simulink model "Validation_Tricopter_Model"  (R2015a)
settings: Solver=ode3  SolverMode=SingleTasking  StartTime=0.0  StopTime=20  FixedStep=T_sim  RelTol=1e-3
PreLoadFcn:
  | LoadLibraries
values from neighbouring files (symbols this model uses):
  a = 10.26    [SetupComplete.m]
  A_x = 0.015    [SetupComplete.m]
  A_y = A_x    (= 0.015)    [SetupComplete.m]
  A_z = 0.16    [SetupComplete.m]
  C_d0 = 0.001193    [SetupComplete.m]
  C_x = 1.2    [SetupComplete.m]
  C_y = C_x    (= 1.2)    [SetupComplete.m]
  C_z = 2.2    [SetupComplete.m]
  CG_0 = [0,0,0.02]'    [SetupComplete.m]
  g = 9.81    [SetupComplete.m]
  h = 0.08    [SetupComplete.m]
  h_FA = 0.02    [SetupComplete.m]
  h_M = 0.064    [SetupComplete.m]
  I_BAC_0 = [ Ix,0,Ixz;0,Iy,0;Ixz,0,Iz]    [SetupComplete.m]
  I_prop = 1/4*M_eq*R^2*diag([1,1,2])    [SetupComplete.m]
  I_tube = [1/2*M_tube*R_tube_eq^2,0,  0  ;           0 ,1/3*M_tube*l_arm^2,0;             0  ,0,1/3*M_tube*l_arm^2]    [SetupComplete.m]
  Initial_Omegas = [1;1;1]*Omega_hover    [Run3Copter.m]
  J_FA = I_prop(1,1) + m_prop*h^2  + m_FA*h_FA^2 + m_M*h_M^2    [SetupComplete.m]
  J_T = J_m+1/2*M_eq*R^2    (= 2.000642e-05)    [SetupComplete.m]
  Ki = lqi(LM_4DOF_aug, Q,R)    [robust_controller.m]
  l = 0.3450    (= 0.345)    [NDI_components.m]    (also in SetupComplete.m; robust_controller.m)
  l_arm = 0.264    [SetupComplete.m]
  m = 3.51    [SetupComplete.m]
  m_0 = 2.61    [SetupComplete.m]
  m_FA = 0.02    [SetupComplete.m]
  m_M = 0.300    (= 0.3)    [SetupComplete.m]
  m_prop = 0.02    [SetupComplete.m]
  R = 0.1778    [SetupComplete.m]    (also in robust_controller.m = eye(4))
  rho = 1.15    [SetupComplete.m]
  sigma = b*c/(pi*R)    (= 0.107416159567)    [SetupComplete.m]
  T_sim = 0.01    [Run3Copter.m]
  theta_0 = 0.38397    [SetupComplete.m]
  theta_1 = -0.2967    [SetupComplete.m]
  trim_simplemodel = [0.589627915568 -2.20656039197 0 0.588313336084 0 0 0.588313330414 0 0]    [trimvalues.mat]
  V_4DOF_last = [0.0122475086001 0.00870447045314 -0.0292257707267 -0.0198753669721 -0.00290766514824 -0.0269511839788 0.0344308792695 -0.0305235710433 -0.0274078219028 -0.0329291952852 -0.0272335702183 -0.00643013158961 ... (1500 elements, 50x30)]    [NN_c_weights.mat]
  v_i0 = sqrt( 1/3*m*g/(2*rho*pi*R^2)  )    [SetupComplete.m]
  W_4DOF_last = [0.0132359246225 -0.0402459595001 -0.0221501781133 0.0046881519205 0.0457506835434 0.0464888535199 -0.0342386918322 0.0470592781761 0.0457166948243 -0.00146243512772 0.0300280468889 -0.0358113661373 ... (204 elements, 4x51)]    [NN_c_weights.mat]
undefined symbols (not defined in the file or in its folder): DOWN_0, EAST_0, Motor, NORTH_0, P_0, Prop, Q_0, R_0, sigmatest, U_0, V_0, v_i_adim, Vx_adim, Vz_adim, W_0
undefined symbols (not defined in the file): Initial_Torques, Rotation_sign, Tau_motors
libraries: simulink x66, XXCopter x32, vrlib x26, simulink_extras x6, Adaptive_FaultTolerantControl x6, qcatlib x4, dspinverses x4, lib_controller x4, aerolib6dofsys x3, aerolibtransform2 x3, aerolib6dof2 x1
(part 11 of 11)

== matlab function Validation_Tricopter_Model/3 Copter Complete/Arms Dynamics: Forces and Moments/4 DOF Arms Dynamics: Forces and Moments1/4 DOF Arms Dynamics: Forces and Moments1/Arm Dynamics/Gyroscopic Moments/Arm Inertia1 ==
  data: T_FAFb input; Arm_axis input; J_Arm output; I_tube parameter; I_prop parameter; h_FA parameter; h_M parameter; m_FA parameter; m_M parameter; m_prop parameter; h parameter
function J_Arm  = Arm_inertia(T_FAFb,Arm_axis, I_tube, I_prop, h_FA, h_M, m_FA, m_M, m_prop, h)


r_FAO=Arm_axis+T_FAFb*[0;0;-h_FA];
r_MO=Arm_axis+T_FAFb*[0;0;-h_M];
r_po=Arm_axis+T_FAFb*[0;0;-h];

I_FA = m_FA*[ r_FAO(2)^2+r_FAO(3)^2,r_FAO(1)*r_FAO(2),r_FAO(1)*r_FAO(3);...
            r_FAO(1)*r_FAO(2), r_FAO(1)^2+r_FAO(3)^2, r_FAO(2)*r_FAO(3);...
            r_FAO(1)*r_FAO(3),r_FAO(2)*r_FAO(3), r_FAO(1)^2+r_FAO(2)^2];
I_M = m_M*[ r_MO(2)^2+r_MO(3)^2,r_MO(1)*r_MO(2),r_MO(1)*r_MO(3);...
            r_MO(1)*r_MO(2), r_MO(1)^2+r_MO(3)^2, r_MO(2)*r_MO(3);...
            r_MO(1)*r_MO(3),r_MO(2)*r_MO(3), r_MO(1)^2+r_MO(2)^2];
I_steiner = m_prop*[ r_po(2)^2+r_po(3)^2,r_po(1)*r_po(2),r_po(1)*r_po(3);...
            r_po(1)*r_po(2), r_po(1)^2+r_po(3)^2, r_po(2)*r_po(3);...
            r_po(1)*r_po(3),r_po(2)*r_po(3), r_po(1)^2+r_po(2)^2];


% J_Arm = T_FAFb*I_prop*T_FAFb'+ I_tube +I_FA+I_M+I_steiner;
J_Arm = T_FAFb*I_prop*T_FAFb' +I_FA+I_M+I_steiner; % Quitamos el tubo ya que es insignificante y hay que calcularlo para cada brazo

== matlab function Validation_Tricopter_Model/Controller/NDI+CA Controller/4DOF ANN+NDI+CA Controller - No massic update/G(X) 4DOF_WPQR ==
  data: gx output size=[4,4]; prev_input input size=[9,1]
function gx = gx(prev_input)
    % Calculates f_hat(x). The expression is calculated in NDI_components
    % x_dot = f(x) + g(x,u)
    %   g(x,u) ~= g(x,u0) + jac(g(x,u), u)(u0) * (u - u0)
    %   g(x,u) ~= h(x,u0) + jac(g(x,u), u)(u0) * u
    % x_dot = f_hat(x) + jac(g(x,u), u) * u
    %   f_hat(x) = f(x) + g(x,u0) - jac(g(x,u), u)(u0) *  u0
    %   g_hat(x) = jac(g(x,u), u)(u0)
    % x_dot = f_hat(x) + g_hat(x) * u
    tau1_0 = prev_input(1);
    eta1_0 = prev_input(2);
    gamma1_0 = prev_input(3);
    tau2_0 = prev_input(4);
    eta2_0 = prev_input(5);
    gamma2_0 = prev_input(6);
    tau3_0 = prev_input(7);
    eta3_0 = prev_input(8);
    gamma3_0 = prev_input(9);
    
    % This matrix was precomputed in NDI_components.m
    % TODO Precompute sines and cosines to improve performance. Some
    % repeated terms can also be precomputed
    
    % Kt = 29.6 Kq = 0.3
    gx = [...
                          -7.379*cos(eta1_0),                                7.379*tau1_0*sin(eta1_0), -7.379,  -7.379;
     0.04359*cos(eta1_0) - 1.541*sin(eta1_0), - 1.541*tau1_0*cos(eta1_0) - 0.04359*tau1_0*sin(eta1_0), -48.41,   48.32;
       43.76*cos(eta1_0) + 1.469*sin(eta1_0),     1.469*tau1_0*cos(eta1_0) - 43.76*tau1_0*sin(eta1_0), -21.88,  -21.88;
       26.0*sin(eta1_0) - 0.8729*cos(eta1_0),     26.0*tau1_0*cos(eta1_0) + 0.8729*tau1_0*sin(eta1_0),  1.997, -0.2515];
 
% Kt = 15 Kq = 0.07
%                        -4.274*cos(eta1_0),                                 4.274*tau1_0*sin(eta1_0), -4.274,  -4.274;
%  0.01017*cos(eta1_0) - 0.8926*sin(eta1_0), - 0.8926*tau1_0*cos(eta1_0) - 0.01017*tau1_0*sin(eta1_0), -28.02,    28.0;
%    25.34*cos(eta1_0) + 0.3428*sin(eta1_0),     0.3428*tau1_0*cos(eta1_0) - 25.34*tau1_0*sin(eta1_0), -12.67,  -12.67;
%    15.06*sin(eta1_0) - 0.2037*cos(eta1_0),     15.06*tau1_0*cos(eta1_0) + 0.2037*tau1_0*sin(eta1_0), 0.8549, -0.4475];

== matlab function Validation_Tricopter_Model/Controller/NDI+CA Controller/4DOF ANN+NDI+CA Controller - No massic update/Adaptive NN/Crossed NN/Cross NN ==
  data: X_bar input size=[30,1]; v_ad_comp output size=4; e input size=6; P input size=[6,6]; B input size=[6,4]; learning_rate input size=1; Reg_param input size=2; W input size=[4,51]; V input size=[50,30]; v_ad output size=4; Z_norm_unit output size=1; T_sim parameter size=1; W_update output size=[4,51]; V_update output size=[50,30]
function [v_ad_comp,v_ad,Z_norm_unit,W_update,V_update]  = Cross_NN(X_bar,e, P, B,learning_rate,Reg_param,W,V,T_sim)

%% Compute prelimiary parameters 
zeta= e'*P*B;

%% Feedforward
z = V*X_bar;
s=sigmoid(V*X_bar);

sigma = [1 ; s ];
% v_ad = W*sigma;

sigma_grad = (sigma.*(ones(size(sigma))-sigma));

%% Compute the gradients or adaptation laws
Gamma_w= learning_rate; % W learnign rate
Gamma_v= learning_rate; %V learning rate
lambda_v = Reg_param(1);
lambda_w = Reg_param(2);

V_dot=zeros(size(V));
W_dot=zeros(size(W));

W_dot= -Gamma_w*(  (sigma - sigma_grad.*[1;z] )*zeta  )';
W_dot(:,2:end)= W_dot(:,2:end) - Gamma_w*lambda_w*norm(zeta)*(W(:,2:end));

M = W'*zeta'.*sigma_grad ;
V_dot= -Gamma_v*( M(2:end)*X_bar'  );
V_dot(:,2:end)= V_dot(:,2:end) - Gamma_v*lambda_v*norm(zeta).*V(:,2:end);

% % % % Other way: Based on notes of Andrew NG
% % % 
% % % delta2=W'*zeta'.*sigma_grad;
% % % 
% % % V_dot = - Gamma_v*( delta2(2:end)*X_bar');
% % % V_dot(:,2:end)= V_dot(:,2:end) - Gamma_v*lambda*norm(zeta).*V(:,2:end);
% % % 
% % % W_dot = - Gamma_w*( sigma*zeta)';
% % % W_dot(:,2:end)= W_dot(:,2:end) - Gamma_w*lambda*norm(zeta)*(W(:,2:end));

%% Adaptation scalled with loop time
W_update = W + T_sim*W_dot;
V_update = V + T_sim*V_dot;

%% Re-compute v_ad
s=sigmoid(V_update*X_bar);

sigma = [1 ; s(:,1) ];
v_ad = W_update*sigma;

%% Compute v_ad_comp (add robustifying terms)
Z = [ V,zeros(size(V,1),size(W,2));
    zeros(size(W,1),size(V,2)),W];
    
Z_norm = norm(Z,'fro');
% Z_max = 2*min(size(W,1),size(W,2) )*min(size(V,1),size(V,2));
Z_max = 1;
Z_norm_unit = Z_norm;

% K_r0= 0.02;
% K_r1= 0;
K_r0= 1;
K_r1= 1;

v_r0 = -K_r0*zeta';
v_r1 = -K_r1*(Z_norm+Z_max)*zeta';

v_ad_comp = v_ad + v_r1 +v_r0;
end

== matlab function Validation_Tricopter_Model/Controller/NDI+CA Controller/4DOF ANN+NDI+CA Controller - No massic update/Rotational Kinematics1 ==
  data: PQR input size=3; Eulerdot output size=3; Euler input size=3
function Eulerdot = rot_kin(PQR,Euler)
%solves rotational kinematic equations
Phi = Euler(1);
Theta = Euler(2);
Psi = Euler(3);
A = [1 sin(Phi)*tan(Theta) cos(Phi)*tan(Theta);
     0 cos(Phi) -sin(Phi);
     0 sin(Phi)*sec(Theta) cos(Phi)*sec(Theta)];
Eulerdot = A*PQR;
end

== matlab function Validation_Tricopter_Model/Controller/NDI+CA Controller/4DOF ANN+NDI+CA Controller - No massic update/Sigmoid /MATLAB Function ==
  data: u input; y output; a input
function y = sigmoid_a(u,a)

y = 2.0 ./ (1.0 + exp(-a*u(:)))-1;

== matlab function Validation_Tricopter_Model/3 Copter Simplified1/6dof Eqs of motion/Accelerometer meas ==
  data: Vb input; omega input; omega_dot input; Ab input; A_s output; r_sens parameter
function A_s  = AcellMeas(Vb,omega,omega_dot,Ab, r_sens)




A_s =  Ab + cross(omega,Vb) + cross(omega, cross(omega,r_sens)) +cross(omega_dot,r_sens)  ;

== matlab function Validation_Tricopter_Model/3 Copter Simplified1/6dof Eqs of motion/Position Eqs ==
  data: A_b output; Vb input; omega input; omega_dot input; Forces input; m input; CG input
function A_b  = PositionEqs(Vb,omega,omega_dot, Forces,m, CG)



 
A_b =  1/m*( Forces ) - cross(omega,Vb) - cross(omega, cross(omega,CG)) -cross(omega_dot,CG)  ;

== matlab function Validation_Tricopter_Model/3 Copter Simplified1/6dof Eqs of motion/Rotational eqs ==
  data: omega_dot output; omega_b input; Moments input; I_BAC input
function omega_dot  = Rotational_Eq(omega_b,Moments, I_BAC)



omega_dot =  I_BAC\( Moments - cross(omega_b,I_BAC*omega_b)  );

== matlab function Validation_Tricopter_Model/3 Copter Simplified1/6dof Eqs of motion/SVFI_to_SVFb ==
  data: X_e input; V_e input; X_e_out output; V_b output; omega_b output; Euler_Ang input; Euler_Ang_Dot input; q output
function [X_e_out,V_b, omega_b ,q]=SVFI_to_SVFb(X_e,V_e, Euler_Ang,Euler_Ang_Dot)

xp=V_e(1);
yp=V_e(2);
zp=V_e(3);

phi=Euler_Ang(1);
theta=Euler_Ang(2);
psi=Euler_Ang(3);
phip=Euler_Ang_Dot(1);
thetap=Euler_Ang_Dot(2);
psip=Euler_Ang_Dot(3);

%%
X_e_out=X_e;

q = QuaternionfromEuler(phi,theta,psi); 



HamOut=HamiltonProduct([q(1);-q(2);-q(3);-q(4)],HamiltonProduct([0;xp;yp;zp],[q(1);q(2);q(3);q(4)]) );% q* . v . q
V_b=HamOut(2:4);

omega_b=[phip-psip*sin(theta)  ;
         thetap*cos(phi)+psip*cos(theta)*sin(phi);
            -thetap*sin(phi)+psip*cos(theta)*cos(phi)  ];% Ya que es solo una operacion aislada utilizaremos la ecuaciones con rel trigonometricas
end
function [q]=QuaternionfromEuler(phi,theta,psi)
% options=optimset('MaxFunEvals',3000);
% q=fsolve(@QUATERNIONEULER,[0.6,0.4,0.5,0.4]); % Hay que acertar con los angulos poniendo diferentes valores iniciales del quaternion
%     function F=QUATERNIONEULER(q)
%         F=[ tan(phi)-(2*q(3)*q(4)-2*q(1)*q(2))/(2*q(1)^2+2*q(4)^2-1)  ;
%             sin(-theta)-2*q(2)*q(4)-2*q(1)*q(3);
%             tan(psi)-(2*q(2)*q(3)-2*q(1)*q(4))/(2*q(1)^2+2*q(2)^2-1);
%             q(1)^2+q(2)^2+q(3)^2+q(4)^2-1];
%     end  % Este algoritmo da q* !!!!!

q=[ cos(psi/2)*cos(theta/2)*cos(phi/2)+ sin(psi/2)*sin(theta/2)*sin(phi/2) ;
      cos(psi/2)*cos(theta/2)*sin(phi/2)- sin(psi/2)*sin(theta/2)*cos(phi/2) ;
       cos(psi/2)*sin(theta/2)*cos(phi/2)+ sin(psi/2)*cos(theta/2)*sin(phi/2)   ;
        sin(psi/2)*cos(theta/2)*cos(phi/2)- cos(psi/2)*sin(theta/2)*sin(phi/2)      ]; % Esto nos da q !!!
end

== matlab function Validation_Tricopter_Model/3 Copter Simplified1/6dof Eqs of motion/SV_F_b_to_SV_FI ==
  data: V_b input; q_dot input; q input; V_e output; euler output; euler_dot output
function [V_e,euler,euler_dot]   = SV_F_b_to_SV_FI(  V_b, q_dot,q)

xp=V_b(1);
yp=V_b(2);
zp=V_b(3);

%% Velocity and position in Earth Frame   q . v . q*

SolProd=HamiltonProduct([q(1);q(2);q(3);q(4)],HamiltonProduct([0;xp;yp;zp],[q(1);-q(2);-q(3);-q(4)]) );
V_e=SolProd(2:4);

%% Actitud en Angulos de Euler y sus derivadas. 
euler=[0,0,0]';
euler(1) = atan2(2*q(3)*q(4)+2*q(1)*q(2),2*q(1)^2+2*q(4)^2-1 ); % phi
euler(2) = -asin( 2*q(2)*q(4)-2*q(1)*q(3) ); %  theta
euler(3) = atan2( 2*q(2)*q(3)+2*q(1)*q(4),2*q(1)^2+2*q(2)^2-1 ); %  psi

euler_dot=[0,0,0]';
euler_dot(1,1) = 2/(1+( (2*q(3)*q(4)+2*q(1)*q(2))/(2*q(1)^2+2*q(4)^2-1)  )^2)*[ -(2*q(1)^2*q(2)+ 4*q(1)*q(3)*q(4)-2*q(2)*q(4)^2+q(2))  ,  q(1)*(2*q(1)^2+2*q(4)^2-1)  ,  q(4)*(2*q(1)^2+2*q(4)^2-1)  ,  -(-2*q(1)^2*q(3) +4*q(1)*q(2)*q(4)+2*q(3)*q(4)^2+q(3) ) ]*q_dot.* 1/(2*q(1)^2+2*q(4)^2-1)^2; % Derivada de phi
euler_dot(2,1) = -2/( sqrt(1-4*(q(2)*q(4)-q(1)*q(3))^2)  )*[-q(3),q(4),-q(1),q(2)]*q_dot;  % Theta prima
euler_dot(3,1) = 2/(1+( (2*q(2)*q(3)+2*q(1)*q(4))/(2*q(1)^2+2*q(2)^2-1)  )^2)*[  -(2*q(1)^2*q(4)+4*q(1)*q(2)*q(3)-2*q(2)^2*q(4)+q(4)  ) , 1/2*(q(3)*(4*q(1)^2-4*q(2)^2-2)-8*q(1)*q(2)*q(4) )  ,  q(2)*(2*q(1)^2+2*q(2)^2-1)  , q(1)*(2*q(1)^2+2*q(2)^2-1) ]*q_dot.*1/(2*q(1)^2+2*q(2)^2-1)^2;  % Psi prima



end

== matlab function Validation_Tricopter_Model/3 Copter Simplified1/6dof Eqs of motion/q_dot/Quaternion_dot ==
  data: omega_b input; q_dot output; q input
function q_dot = Quaternion_dot(omega_b,q)


q_dot = 1/2*HamiltonProduct(q,[0;omega_b]);

== matlab function Validation_Tricopter_Model/3 Copter Simplified1/MATLAB Function ==
  data: input input; Tbody_ext output; Mbody_ext output; Kt input; Kq input; v_body input; omega_body input
function [Tbody_ext, Mbody_ext] = fcn(input, Kt, Kq, v_body, omega_body)
    tau1 = input(1);
    eta1 = input(2);
    gamma1 = input(3);
    tau2 = input(4);
    eta2 = input(5);
    gamma2 = input(6);
    tau3 = input(7);
    eta3 = input(8);
    gamma3= input(9);
    U = v_body(1);
    V = v_body(2);
    W = v_body(3);
    P = omega_body(1);
    Q = omega_body(2);
    R = omega_body(3);

Tbody_ext = [...
           - Kt*tau1*sin(gamma1) - Kt*tau2*cos(gamma2)*sin(eta2) - Kt*tau3*cos(gamma3)*sin(eta3);
                       Kt*tau2*sin(gamma2) + Kt*tau3*sin(gamma3) + Kt*tau1*cos(gamma1)*sin(eta1);
 - Kt*tau1*cos(eta1)*cos(gamma1) - Kt*tau2*cos(eta2)*cos(gamma2) - Kt*tau3*cos(eta3)*cos(gamma3)];
 

Mbody_ext = [...
                                                                                                                  (5382319726372233*Kt*tau3*cos(eta3)*cos(gamma3))/18014398509481984 - (5382319726372233*Kt*tau2*cos(eta2)*cos(gamma2))/18014398509481984 - Kq*tau1*sin(gamma1) + Kq*tau2*cos(gamma2)*sin(eta2) + Kq*tau3*cos(gamma3)*sin(eta3);
                                                                                                                                           (69*Kt*tau1*cos(eta1)*cos(gamma1))/200 - Kq*tau3*sin(gamma3) - Kq*tau2*sin(gamma2) - (69*Kt*tau2*cos(eta2)*cos(gamma2))/400 - (69*Kt*tau3*cos(eta3)*cos(gamma3))/400 + Kq*tau1*cos(gamma1)*sin(eta1);
 Kq*tau2*cos(eta2)*cos(gamma2) - (69*Kt*tau3*sin(gamma3))/400 - Kq*tau1*cos(eta1)*cos(gamma1) - (69*Kt*tau2*sin(gamma2))/400 + Kq*tau3*cos(eta3)*cos(gamma3) + (69*Kt*tau1*cos(gamma1)*sin(eta1))/200 + (5382319726372233*Kt*tau2*cos(gamma2)*sin(eta2))/18014398509481984 - (5382319726372233*Kt*tau3*cos(gamma3)*sin(eta3))/18014398509481984];

== matlab function Validation_Tricopter_Model/3 Copter Complete/Arms Dynamics: Forces and Moments/9 DOF Arms Dynamics: Forces and Moments/9 DOF Arms Dynamics: Forces and Moments/Arm Dynamics1/Arms Kinematics/DCM Arm ==
  data: arm_no input; eta input; T_Fb_FA output; gamma input
function T_Fb_FA = DCM_Arm(arm_no,eta, gamma)
    T_Fb_FA = [cos(eta),0,-sin(eta) ;...
            sin(eta)*sin(gamma),cos(gamma),cos(eta)*sin(gamma);...
            sin(eta)*cos(gamma),-sin(gamma),cos(eta)*cos(gamma)];

== matlab function Validation_Tricopter_Model/3 Copter Complete/Arms Dynamics: Forces and Moments/9 DOF Arms Dynamics: Forces and Moments/9 DOF Arms Dynamics: Forces and Moments/Arm Dynamics2/Arms Kinematics/DCM Arm ==
  data: arm_no input; eta input; T_Fb_FA output; gamma input
function T_Fb_FA = DCM_Arm(arm_no,eta, gamma)
    T_Fb_FA = [cos(eta),0,-sin(eta) ;...
            sin(eta)*sin(gamma),cos(gamma),cos(eta)*sin(gamma);...
            sin(eta)*cos(gamma),-sin(gamma),cos(eta)*cos(gamma)];

== matlab function Validation_Tricopter_Model/Controller/NDI+CA Controller/4DOF ANN+NDI+CA Controller - No massic update/F(X) ==
  data: fx output size=[4,1]; prev_input input size=[9,1]; gforce_body input size=[3,1]; omega_body input size=[3,1]; v_body input size=[3,1]
function fx = fx(prev_input, gforce_body, omega_body, v_body)
    % Calculates f_hat(x). The expression is calculated in NDI_components
    % x_dot = f(x) + g(x,u)
    %   g(x,u) ~= g(x,u0) + jac(g(x,u), u)(u0) * (u - u0)
    %   g(x,u) ~= h(x,u0) + jac(g(x,u), u)(u0) * u
    % x_dot = f_hat(x) + jac(g(x,u), u) * u
    %   f_hat(x) = f(x) + g(x,u0) - jac(g(x,u), u)(u0) *  u0
    %   g_hat(x) = jac(g(x,u), u)(u0)
    % x_dot = f_hat(x) + g_hat(x) * u
    tau1_0 = prev_input(1);
    eta1_0 = prev_input(2);
    gamma1_0 = prev_input(3);
    tau2_0 = prev_input(4);
    eta2_0 = prev_input(5);
    gamma2_0 = prev_input(6);
    tau3_0 = prev_input(7);
    eta3_0 = prev_input(8);
    gamma3_0 = prev_input(9);
    Gx =  gforce_body(1);
    Gy =  gforce_body(2);
    Gz =  gforce_body(3);
    U = v_body(1);
    V = v_body(2);
    W = v_body(3);
    P = omega_body(1);
    Q = omega_body(2);
    R = omega_body(3);

    % This matrix was precomputed in NDI_components.m
    % TODO Precompute sines and cosines to improve performance. Some
    % repeated terms can also be precomputed
    
 % Kt = 29.6 Kq = 0.3
 fx = [... 
                    - 0.0015*P^2 - 1.0*V*P - 0.0015*Q^2 + U*Q + 0.2849*Gz - 7.379*eta1_0*tau1_0*sin(eta1_0);
              1.541*eta1_0*tau1_0*cos(eta1_0) - 0.8756*Q*R - 0.0436*P*Q + 0.04359*eta1_0*tau1_0*sin(eta1_0);
 0.03918*P^2 + 0.9007*P*R - 0.03918*R^2 - 1.469*eta1_0*tau1_0*cos(eta1_0) + 43.76*eta1_0*tau1_0*sin(eta1_0);
                0.0436*Q*R - 0.1269*P*Q - 26.0*eta1_0*tau1_0*cos(eta1_0) - 0.8729*eta1_0*tau1_0*sin(eta1_0)];    
 
% Kt = 15 Kq = 0.07
%                          - 0.0015*P^2 - 1.0*V*P - 0.0015*Q^2 + 1.0*U*Q + 0.2849*Gz - 4.2735*eta1_0*tau1_0*sin(eta1_0);
%                   0.89255*eta1_0*tau1_0*cos(eta1_0) - 0.87555*Q*R - 0.043605*P*Q + 0.010171*eta1_0*tau1_0*sin(eta1_0);
%      0.039179*P^2 + 0.90066*P*R - 0.039179*R^2 - 0.34281*eta1_0*tau1_0*cos(eta1_0) + 25.344*eta1_0*tau1_0*sin(eta1_0);
%                      0.043605*Q*R - 0.12686*P*Q - 15.06*eta1_0*tau1_0*cos(eta1_0) - 0.20367*eta1_0*tau1_0*sin(eta1_0)];

== matlab function Validation_Tricopter_Model/Controller/NDI+CA Controller/4DOF ANN+NDI+CA Controller - No massic update/Rotational Kinematics2 ==
  data: PQR output size=3; Eulerdot input size=3; Euler input size=3
function PQR = rot_kin(Eulerdot,Euler)
%solves rotational kinematic equations
Phi = Euler(1);
Theta = Euler(2);
Psi = Euler(3);
A = [1 sin(Phi)*tan(Theta) cos(Phi)*tan(Theta);
     0 cos(Phi) -sin(Phi);
     0 sin(Phi)*sec(Theta) cos(Phi)*sec(Theta)];
PQR = A'*Eulerdot;
end

== matlab function Validation_Tricopter_Model/Controller/NDI+CA Controller/4DOF ANN+NDI+CA Controller - No massic update Aero Uncertainty Variant/Rotational Kinematics2 ==
  data: PQR output size=3; Eulerdot input size=3; Euler input size=3
function PQR = rot_kin(Eulerdot,Euler)
%solves rotational kinematic equations
Phi = Euler(1);
Theta = Euler(2);
Psi = Euler(3);
A = [1 sin(Phi)*tan(Theta) cos(Phi)*tan(Theta);
     0 cos(Phi) -sin(Phi);
     0 sin(Phi)*sec(Theta) cos(Phi)*sec(Theta)];
PQR = A'*Eulerdot;
end

== matlab function Validation_Tricopter_Model/Controller/NDI+CA Controller/4DOF ANN+NDI+CA Controller - No massic update Aero Uncertainty Variant/Sigmoid /MATLAB Function ==
  data: u input; y output; a input
function y = sigmoid_a(u,a)

y = 2.0 ./ (1.0 + exp(-a*u(:)))-1;

== matlab function Validation_Tricopter_Model/Controller/NDI+CA Controller/4DOF ANN+NDI+CA Controller - No massic update/Adaptive NN/Crossed NN/MATLAB Function ==
  data: P1 input; P output; P2 input; P3 input; P4 input
function P = fcn(P1,P2,P3,P4)
%#codegen

P = blkdiag(P1,P2,P3,P4);

== matlab function Validation_Tricopter_Model/Controller/NDI+CA Controller/4DOF ANN+NDI+CA Controller - No massic update/Adaptive NN/Crossed NN/MATLAB Function1 ==
  data: P1 input; P output; P2 input; P3 input; P4 input
function P = fcn(P1,P2,P3,P4)
%#codegen

P = blkdiag(P1,P2,P3,P4);

== matlab function Validation_Tricopter_Model/Controller/NDI+CA Controller/4DOF ANN+NDI+CA Controller - No massic update/Adaptive NN/Crossed NN/MATLAB Function2 ==
  data: P1 input; P output; P2 input; P3 input; P4 input
function P = fcn(P1,P2,P3,P4)
%#codegen

P = [P1;P2;P3;P4];

== matlab function Validation_Tricopter_Model/Controller/NDI+CA Controller/4DOF NDI+CA Controller - No massic update/F(X)1 ==
  data: fx output size=[4,1]; prev_input input size=[9,1]; gforce_body input size=[3,1]; omega_body input size=[3,1]; v_body input size=[3,1]
function fx = fx(prev_input, gforce_body, omega_body, v_body)
    % Calculates f_hat(x). The expression is calculated in NDI_components
    % x_dot = f(x) + g(x,u)
    %   g(x,u) ~= g(x,u0) + jac(g(x,u), u)(u0) * (u - u0)
    %   g(x,u) ~= h(x,u0) + jac(g(x,u), u)(u0) * u
    % x_dot = f_hat(x) + jac(g(x,u), u) * u
    %   f_hat(x) = f(x) + g(x,u0) - jac(g(x,u), u)(u0) *  u0
    %   g_hat(x) = jac(g(x,u), u)(u0)
    % x_dot = f_hat(x) + g_hat(x) * u
    tau1_0 = prev_input(1);
    eta1_0 = prev_input(2);
    gamma1_0 = prev_input(3);
    tau2_0 = prev_input(4);
    eta2_0 = prev_input(5);
    gamma2_0 = prev_input(6);
    tau3_0 = prev_input(7);
    eta3_0 = prev_input(8);
    gamma3_0 = prev_input(9);
    Gx =  gforce_body(1);
    Gy =  gforce_body(2);
    Gz =  gforce_body(3);
    U = v_body(1);
    V = v_body(2);
    W = v_body(3);
    P = omega_body(1);
    Q = omega_body(2);
    R = omega_body(3);

    % This matrix was precomputed in NDI_components.m
    % TODO Precompute sines and cosines to improve performance. Some
    % repeated terms can also be precomputed
    
 % Kt = 29.6 Kq = 0.3
 fx = [... 
                    - 0.0015*P^2 - 1.0*V*P - 0.0015*Q^2 + U*Q + 0.2849*Gz - 7.379*eta1_0*tau1_0*sin(eta1_0);
              1.541*eta1_0*tau1_0*cos(eta1_0) - 0.8756*Q*R - 0.0436*P*Q + 0.04359*eta1_0*tau1_0*sin(eta1_0);
 0.03918*P^2 + 0.9007*P*R - 0.03918*R^2 - 1.469*eta1_0*tau1_0*cos(eta1_0) + 43.76*eta1_0*tau1_0*sin(eta1_0);
                0.0436*Q*R - 0.1269*P*Q - 26.0*eta1_0*tau1_0*cos(eta1_0) - 0.8729*eta1_0*tau1_0*sin(eta1_0)];    
 
% Kt = 15 Kq = 0.07
%                          - 0.0015*P^2 - 1.0*V*P - 0.0015*Q^2 + 1.0*U*Q + 0.2849*Gz - 4.2735*eta1_0*tau1_0*sin(eta1_0);
%                   0.89255*eta1_0*tau1_0*cos(eta1_0) - 0.87555*Q*R - 0.043605*P*Q + 0.010171*eta1_0*tau1_0*sin(eta1_0);
%      0.039179*P^2 + 0.90066*P*R - 0.039179*R^2 - 0.34281*eta1_0*tau1_0*cos(eta1_0) + 25.344*eta1_0*tau1_0*sin(eta1_0);
%                      0.043605*Q*R - 0.12686*P*Q - 15.06*eta1_0*tau1_0*cos(eta1_0) - 0.20367*eta1_0*tau1_0*sin(eta1_0)];

== matlab function Validation_Tricopter_Model/Controller/NDI+CA Controller/4DOF NDI+CA Controller - No massic update/G(X) 4DOF_WPQR1 ==
  data: gx output size=[4,4]; prev_input input size=[9,1]
function gx = gx(prev_input)
    % Calculates f_hat(x). The expression is calculated in NDI_components
    % x_dot = f(x) + g(x,u)
    %   g(x,u) ~= g(x,u0) + jac(g(x,u), u)(u0) * (u - u0)
    %   g(x,u) ~= h(x,u0) + jac(g(x,u), u)(u0) * u
    % x_dot = f_hat(x) + jac(g(x,u), u) * u
    %   f_hat(x) = f(x) + g(x,u0) - jac(g(x,u), u)(u0) *  u0
    %   g_hat(x) = jac(g(x,u), u)(u0)
    % x_dot = f_hat(x) + g_hat(x) * u
    tau1_0 = prev_input(1);
    eta1_0 = prev_input(2);
    gamma1_0 = prev_input(3);
    tau2_0 = prev_input(4);
    eta2_0 = prev_input(5);
    gamma2_0 = prev_input(6);
    tau3_0 = prev_input(7);
    eta3_0 = prev_input(8);
    gamma3_0 = prev_input(9);
    
    % This matrix was precomputed in NDI_components.m
    % TODO Precompute sines and cosines to improve performance. Some
    % repeated terms can also be precomputed
    
    % Kt = 29.6 Kq = 0.3
    gx = [...
                          -7.379*cos(eta1_0),                                7.379*tau1_0*sin(eta1_0), -7.379,  -7.379;
     0.04359*cos(eta1_0) - 1.541*sin(eta1_0), - 1.541*tau1_0*cos(eta1_0) - 0.04359*tau1_0*sin(eta1_0), -48.41,   48.32;
       43.76*cos(eta1_0) + 1.469*sin(eta1_0),     1.469*tau1_0*cos(eta1_0) - 43.76*tau1_0*sin(eta1_0), -21.88,  -21.88;
       26.0*sin(eta1_0) - 0.8729*cos(eta1_0),     26.0*tau1_0*cos(eta1_0) + 0.8729*tau1_0*sin(eta1_0),  1.997, -0.2515];
 
% Kt = 15 Kq = 0.07
%                        -4.274*cos(eta1_0),                                 4.274*tau1_0*sin(eta1_0), -4.274,  -4.274;
%  0.01017*cos(eta1_0) - 0.8926*sin(eta1_0), - 0.8926*tau1_0*cos(eta1_0) - 0.01017*tau1_0*sin(eta1_0), -28.02,    28.0;
%    25.34*cos(eta1_0) + 0.3428*sin(eta1_0),     0.3428*tau1_0*cos(eta1_0) - 25.34*tau1_0*sin(eta1_0), -12.67,  -12.67;
%    15.06*sin(eta1_0) - 0.2037*cos(eta1_0),     15.06*tau1_0*cos(eta1_0) + 0.2037*tau1_0*sin(eta1_0), 0.8549, -0.4475];

== matlab function Validation_Tricopter_Model/Controller/NDI+CA Controller/4DOF NDI+CA Controller - No massic update/Rotational Kinematics ==
  data: PQR output; Eulerdot input; Euler input
function PQR = rot_kin(Eulerdot,Euler)
%solves rotational kinematic equations
Phi = Euler(1);
Theta = Euler(2);
Psi = Euler(3);
A = [1 sin(Phi)*tan(Theta) cos(Phi)*tan(Theta);
     0 cos(Phi) -sin(Phi);
     0 sin(Phi)*sec(Theta) cos(Phi)*sec(Theta)];
PQR = A'*Eulerdot;
end

== matlab function Validation_Tricopter_Model/3 Copter Complete/Arms Dynamics: Forces and Moments/9 DOF Arms Dynamics: Forces and Moments/9 DOF Arms Dynamics: Forces and Moments/Arm Dynamics1/Gyroscopic Moments/Arm Inertia1 ==
  data: T_FAFb input; Arm_axis input; J_Arm output; I_tube parameter; I_prop parameter; h_FA parameter; h_M parameter; m_FA parameter; m_M parameter; m_prop parameter; h parameter
function J_Arm  = Arm_inertia(T_FAFb,Arm_axis, I_tube, I_prop, h_FA, h_M, m_FA, m_M, m_prop, h)


r_FAO=Arm_axis+T_FAFb*[0;0;-h_FA];
r_MO=Arm_axis+T_FAFb*[0;0;-h_M];
r_po=Arm_axis+T_FAFb*[0;0;-h];

I_FA = m_FA*[ r_FAO(2)^2+r_FAO(3)^2,r_FAO(1)*r_FAO(2),r_FAO(1)*r_FAO(3);...
            r_FAO(1)*r_FAO(2), r_FAO(1)^2+r_FAO(3)^2, r_FAO(2)*r_FAO(3);...
            r_FAO(1)*r_FAO(3),r_FAO(2)*r_FAO(3), r_FAO(1)^2+r_FAO(2)^2];
I_M = m_M*[ r_MO(2)^2+r_MO(3)^2,r_MO(1)*r_MO(2),r_MO(1)*r_MO(3);...
            r_MO(1)*r_MO(2), r_MO(1)^2+r_MO(3)^2, r_MO(2)*r_MO(3);...
            r_MO(1)*r_MO(3),r_MO(2)*r_MO(3), r_MO(1)^2+r_MO(2)^2];
I_steiner = m_prop*[ r_po(2)^2+r_po(3)^2,r_po(1)*r_po(2),r_po(1)*r_po(3);...
            r_po(1)*r_po(2), r_po(1)^2+r_po(3)^2, r_po(2)*r_po(3);...
            r_po(1)*r_po(3),r_po(2)*r_po(3), r_po(1)^2+r_po(2)^2];


% J_Arm = T_FAFb*I_prop*T_FAFb'+ I_tube +I_FA+I_M+I_steiner;
J_Arm = T_FAFb*I_prop*T_FAFb' +I_FA+I_M+I_steiner; % Quitamos el tubo ya que es insignificante y hay que calcularlo para cada brazo

== matlab function Validation_Tricopter_Model/3 Copter Complete/Arms Dynamics: Forces and Moments/9 DOF Arms Dynamics: Forces and Moments/9 DOF Arms Dynamics: Forces and Moments/Arm Dynamics2/Gyroscopic Moments/Arm Inertia1 ==
  data: T_FAFb input; Arm_axis input; J_Arm output; I_tube parameter; I_prop parameter; h_FA parameter; h_M parameter; m_FA parameter; m_M parameter; m_prop parameter; h parameter
function J_Arm  = Arm_inertia(T_FAFb,Arm_axis, I_tube, I_prop, h_FA, h_M, m_FA, m_M, m_prop, h)


r_FAO=Arm_axis+T_FAFb*[0;0;-h_FA];
r_MO=Arm_axis+T_FAFb*[0;0;-h_M];
r_po=Arm_axis+T_FAFb*[0;0;-h];

I_FA = m_FA*[ r_FAO(2)^2+r_FAO(3)^2,r_FAO(1)*r_FAO(2),r_FAO(1)*r_FAO(3);...
            r_FAO(1)*r_FAO(2), r_FAO(1)^2+r_FAO(3)^2, r_FAO(2)*r_FAO(3);...
            r_FAO(1)*r_FAO(3),r_FAO(2)*r_FAO(3), r_FAO(1)^2+r_FAO(2)^2];
I_M = m_M*[ r_MO(2)^2+r_MO(3)^2,r_MO(1)*r_MO(2),r_MO(1)*r_MO(3);...
            r_MO(1)*r_MO(2), r_MO(1)^2+r_MO(3)^2, r_MO(2)*r_MO(3);...
            r_MO(1)*r_MO(3),r_MO(2)*r_MO(3), r_MO(1)^2+r_MO(2)^2];
I_steiner = m_prop*[ r_po(2)^2+r_po(3)^2,r_po(1)*r_po(2),r_po(1)*r_po(3);...
            r_po(1)*r_po(2), r_po(1)^2+r_po(3)^2, r_po(2)*r_po(3);...
            r_po(1)*r_po(3),r_po(2)*r_po(3), r_po(1)^2+r_po(2)^2];


% J_Arm = T_FAFb*I_prop*T_FAFb'+ I_tube +I_FA+I_M+I_steiner;
J_Arm = T_FAFb*I_prop*T_FAFb' +I_FA+I_M+I_steiner; % Quitamos el tubo ya que es insignificante y hay que calcularlo para cada brazo

== matlab function Validation_Tricopter_Model/3 Copter Complete/Arms Dynamics: Forces and Moments/9 DOF Arms Dynamics: Forces and Moments/9 DOF Arms Dynamics: Forces and Moments/Arm Dynamics/Gyroscopic Moments/Arm Inertia1 ==
  data: T_FAFb input; Arm_axis input; J_Arm output; I_tube parameter; I_prop parameter; h_FA parameter; h_M parameter; m_FA parameter; m_M parameter; m_prop parameter; h parameter
function J_Arm  = Arm_inertia(T_FAFb,Arm_axis, I_tube, I_prop, h_FA, h_M, m_FA, m_M, m_prop, h)


r_FAO=Arm_axis+T_FAFb*[0;0;-h_FA];
r_MO=Arm_axis+T_FAFb*[0;0;-h_M];
r_po=Arm_axis+T_FAFb*[0;0;-h];

I_FA = m_FA*[ r_FAO(2)^2+r_FAO(3)^2,r_FAO(1)*r_FAO(2),r_FAO(1)*r_FAO(3);...
            r_FAO(1)*r_FAO(2), r_FAO(1)^2+r_FAO(3)^2, r_FAO(2)*r_FAO(3);...
            r_FAO(1)*r_FAO(3),r_FAO(2)*r_FAO(3), r_FAO(1)^2+r_FAO(2)^2];
I_M = m_M*[ r_MO(2)^2+r_MO(3)^2,r_MO(1)*r_MO(2),r_MO(1)*r_MO(3);...
            r_MO(1)*r_MO(2), r_MO(1)^2+r_MO(3)^2, r_MO(2)*r_MO(3);...
            r_MO(1)*r_MO(3),r_MO(2)*r_MO(3), r_MO(1)^2+r_MO(2)^2];
I_steiner = m_prop*[ r_po(2)^2+r_po(3)^2,r_po(1)*r_po(2),r_po(1)*r_po(3);...
            r_po(1)*r_po(2), r_po(1)^2+r_po(3)^2, r_po(2)*r_po(3);...
            r_po(1)*r_po(3),r_po(2)*r_po(3), r_po(1)^2+r_po(2)^2];


% J_Arm = T_FAFb*I_prop*T_FAFb'+ I_tube +I_FA+I_M+I_steiner;
J_Arm = T_FAFb*I_prop*T_FAFb' +I_FA+I_M+I_steiner; % Quitamos el tubo ya que es insignificante y hay que calcularlo para cada brazo
